simulink model "labor11_Sim"  (R2024a)
settings: Solver=VariableStepAuto  StartTime=0.0  StopTime=20  MaxStep=0.1  RelTol=1e-3
values from neighbouring files (symbols this model uses):
  A = [0 1;-k/m -b/m]    [lab_11.m]    (also in labor11.m)
  B = [0; 1/m]    [lab_11.m]    (also in labor11.m = [0;1/m])
  K = acker(A,B,[sc1 sc2])    [labor11.m]
settings Model: Creator=hallgato  LastModifiedBy=hallgato

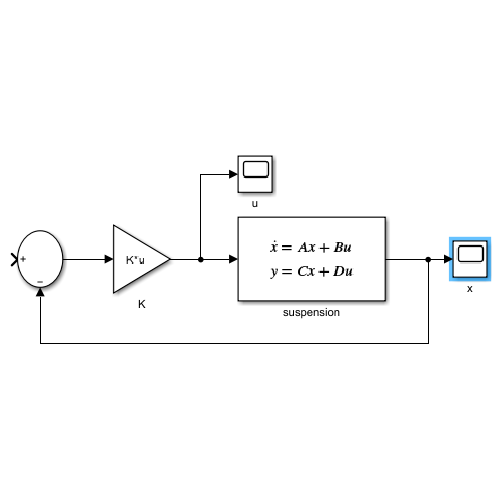
[thumbnail: Simulink's stored preview of the top-level diagram]
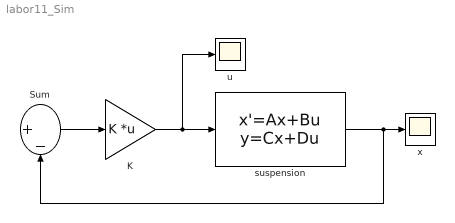
== system labor11_Sim ==
  K : Gain  Gain=K  Multiplication=Matrix(K*u)
  Sum : Sum  Inputs=|+-
  suspension : StateSpace  A=A  B=B  C=eye(2)  D=zeros(2,1)  InitialCondition=[0.1 0]
  u : Scope
  x : Scope
  wires:
  suspension/1 -> Sum/2, x/1
  K/1 -> u/1, suspension/1
  Sum/1 -> K/1
